simulink model "msdMultipleSoln"  (R2024a)
settings: Solver=VariableStepAuto  StartTime=0.0  StopTime=40  RelTol=1e-6
settings Model: Creator=Rocksmithed  LastModifiedBy=vboutrou
settings SolverCC: AlgebraicLoopSolver=TrustRegion
settings DataIOCC: SaveFormat=Array
settings DebuggingCC: UnconnectedInputMsg=warning  UnconnectedOutputMsg=warning  UnconnectedLineMsg=warning
settings HardwareCC: TargetBitPerPointer=64  TargetBitPerSizeT=64  TargetBitPerPtrDiffT=64  TargetLongLongMode=on  TargetIntDivRoundTo=Zero  TargetEndianess=LittleEndian  TargetWordSize=64  TargetHWDeviceType=MATLAB Host  ProdEqTarget=off
settings ModelReferenceCC: EnableRefExpFcnMdlSchedulingChecks=on
settings RTWCC: Description=Rapid Simulation Target  SystemTargetFile=rsim.tlc  TemplateMakefile=rsim_default_tmf  GPUComputeCapability=3.5  DLArmComputeVersion=19.05
settings RSimTargetCC: TargetLangStandard=C99 (ISO)  InstructionSetFMA=off  OptimizeReductions=off  LogToMDFFile=off

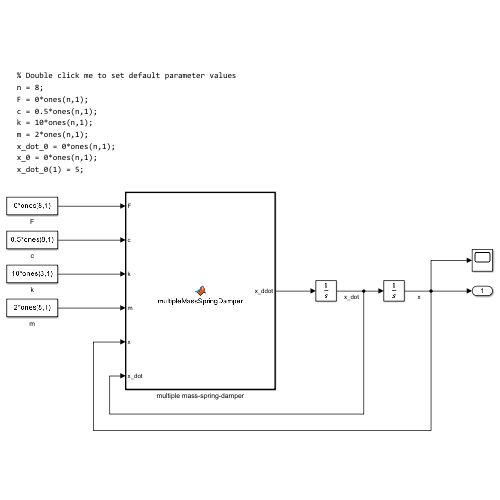
[thumbnail: Simulink's stored preview of the top-level diagram]
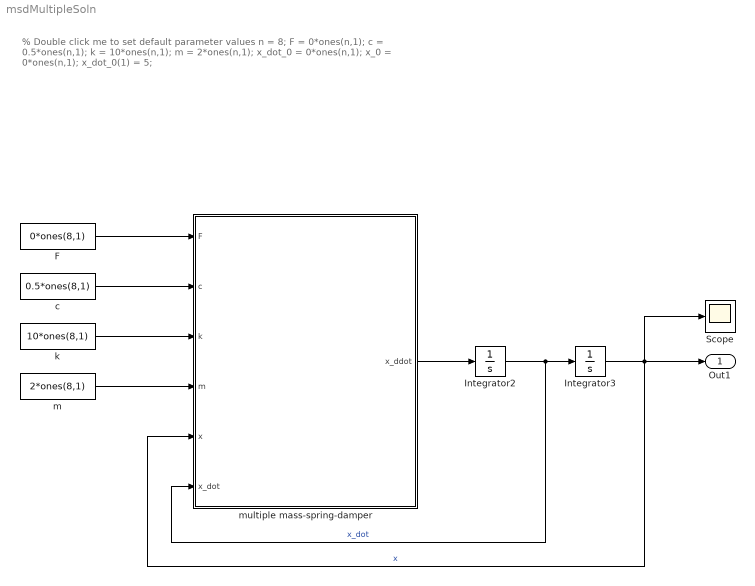
== system msdMultipleSoln ==
  note: % Double click me to set default parameter values
      | n = 8;
      | F = 0*ones(n,1);
      | c = 0.5*ones(n,1);
      | k = 10*ones(n,1);
      | m = 2*ones(n,1);
      | x_dot_0 = 0*ones(n,1);
      | x_0 = 0*ones(n,1);
      | x_dot_0(1) = 5;
  F : Constant  Value=0*ones(8,1)
  Integrator2 : Integrator  InitialCondition=[5;0;0;0;0;0;0;0]
  Integrator3 : Integrator  InitialCondition=0*ones(8,1)
  Scope : Scope
  c : Constant  Value=0.5*ones(8,1)
  k : Constant  Value=10*ones(8,1)
  m : Constant  Value=2*ones(8,1)
  multiple mass-spring-damper : MATLAB Function  TreatAsAtomicUnit=on
  Out1 : Outport
  wires:
  Integrator2/1 -> multiple mass-spring-damper/6(x_dot), Integrator3/1  "x_dot"
  Integrator3/1 -> Out1/1, multiple mass-spring-damper/5(x), Scope/1  "x"
  F/1 -> multiple mass-spring-damper/1(F)
  c/1 -> multiple mass-spring-damper/2(c)
  k/1 -> multiple mass-spring-damper/3(k)
  m/1 -> multiple mass-spring-damper/4(m)
  multiple mass-spring-damper/1(x_ddot) -> Integrator2/1

== matlab function msdMultipleSoln/multiple mass-spring-damper ==
  data: F input; x_ddot output; c input; k input; m input; x input; x_dot input
function x_ddot = multipleMassSpringDamper(F, c, k, m, x, x_dot)
%#codegen

n = 8;

x_ddot = zeros(n,1);

x_ddot(1) = -(-F(1)+c(1).*x_dot(1)+k(1).*x(1)+c(2).*(x_dot(1)-x_dot(2))+k(2).*(x(1)-x(2)))./m(1);
if (n > 2)
    x_ddot(2:n-1) = F(2:n-1) + k(3:n).*( x(3:n) - x(2:n-1) ) + c(3:n).*( x_dot(3:n) - x_dot(2:n-1) )...
                             - k(2:n-1).*( x(2:n-1) - x(1:n-2) ) - c(2:n-1).*( x_dot(2:n-1) - x_dot(1:n-2) );
end
x_ddot(n) = (F(n)-c(n).*(x_dot(n)-x_dot(n-1))-k(n).*(x(n)-x(n-1)))./m(n) ;
